simulink model "flanger"  (R2019a)
settings: Solver=FixedStepDiscrete  StartTime=0.0  StopTime=stop_time  RelTol=1e-3
InitFcn:
  | sm_callback_init
StopFcn:
  | sm_callback_stop
values from neighbouring files (symbols this model uses):
  mp = sm_init_avalon_signals(mp)    [sm_callback_init.m]
libraries: simulink x3, dspsigops x2
settings Model: Creator=Ross  LastModifiedBy=bugsbunny
settings DataIOCC: ReturnWorkspaceOutputs=off
settings OptimizationCC: BlockReduction=off  ConditionallyExecuteInputs=off  DefaultParameterBehavior=Inlined
settings DebuggingCC: ReadBeforeWriteMsg=DisableAll  WriteAfterWriteMsg=DisableAll  WriteAfterReadMsg=DisableAll  AlgebraicLoopMsg=error  MultiTaskDSMMsg=none  SingleTaskRateTransMsg=error  PregeneratedLibrarySubsystemCodeDiagnostic=none  ArithmeticOperatorsInVariantConditions=warning
settings HardwareCC: ProdBitPerPointer=32  ProdBitPerSizeT=32  ProdBitPerPtrDiffT=32  ProdLargestAtomicFloat=None  ProdIntDivRoundTo=Undefined  ProdEndianess=Unspecified  ProdWordSize=32  ProdHWDeviceType=ASIC/FPGA->ASIC/FPGA  TargetBitPerPointer=64  TargetBitPerSizeT=64  TargetBitPerPtrDiffT=64  TargetLongLongMode=on  TargetIntDivRoundTo=Zero  TargetEndianess=LittleEndian  TargetWordSize=64  TargetHWDeviceType=Custom Processor->MATLAB Host Computer  ProdEqTarget=off
settings ModelReferenceCC: UpdateModelReferenceTargets=IfOutOfDate
settings SFSimCC: SFSimEcho=off  SimUseLocalCustomCode=off
settings RTWCC: RTWUseLocalCustomCode=off

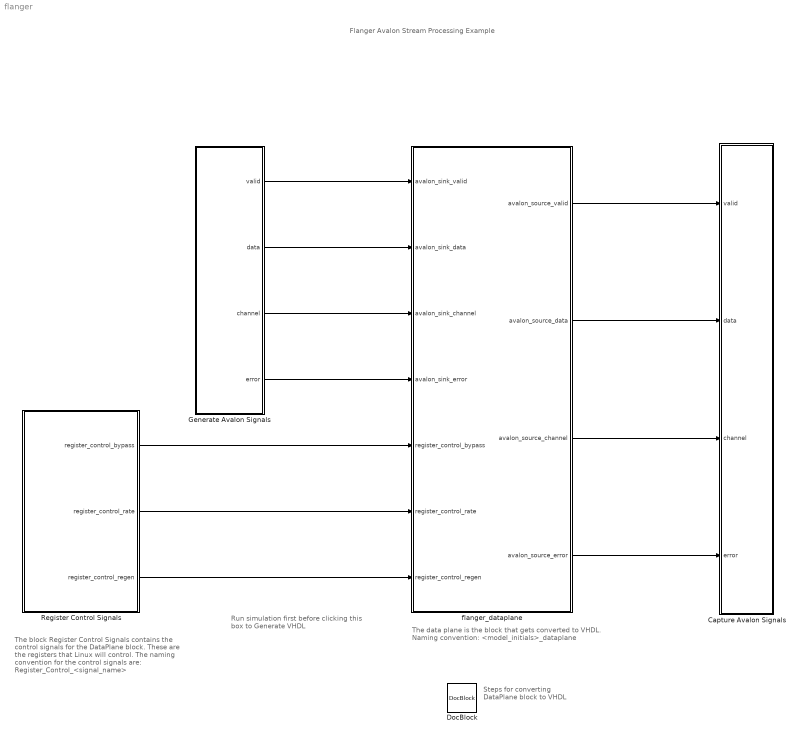
== system flanger ==
  note: The data plane is the block that gets converted to VHDL. Naming convention: <model_initials>_dataplane
  note: Steps for converting
      | DataPlane block
      | to VHDL
  note: Flanger
      | Avalon Stream Processing Example
  note: Run simulation first
      | before clicking this box to
      | Generate VHDL
  note: The block Register Control Signals contains
      | the control signals for the DataPlane block.
      | These are the registers that Linux will control.
      | The naming convention for the control
      | signals are:  Register_Control_<signal_name>
  Capture Avalon Signals : Subsystem
  DocBlock : simulink/Model-Wide Utilities/DocBlock  DocumentType=HTML
  Generate Avalon Signals : Subsystem
  Register Control Signals : Subsystem
  flanger_dataplane : Subsystem  TreatAsAtomicUnit=on
  wires:
  Generate Avalon Signals/2(data) -> flanger_dataplane/2(avalon_sink_data)
  Generate Avalon Signals/1(valid) -> flanger_dataplane/1(avalon_sink_valid)
  Generate Avalon Signals/3(channel) -> flanger_dataplane/3(avalon_sink_channel)
  Generate Avalon Signals/4(error) -> flanger_dataplane/4(avalon_sink_error)
  flanger_dataplane/2(avalon_source_data) -> Capture Avalon Signals/2(data)
  flanger_dataplane/1(avalon_source_valid) -> Capture Avalon Signals/1(valid)
  flanger_dataplane/3(avalon_source_channel) -> Capture Avalon Signals/3(channel)
  flanger_dataplane/4(avalon_source_error) -> Capture Avalon Signals/4(error)
  Register Control Signals/1(register_control_bypass) -> flanger_dataplane/5(register_control_bypass)
  Register Control Signals/2(register_control_rate) -> flanger_dataplane/6(register_control_rate)
  Register Control Signals/3(register_control_regen) -> flanger_dataplane/7(register_control_regen)

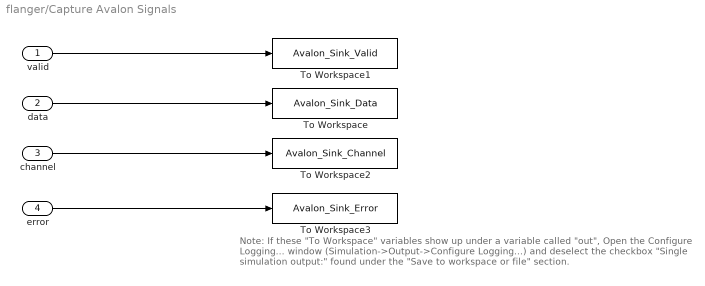
== system flanger/Capture Avalon Signals ==
  note: Note:  If these "To Workspace" variables show up under a variable called "out",
      | Open the Configure Logging... window (Simulation->Output->Configure Logging...)
      | and deselect the checkbox "Single simulation output:" found under the "Save to workspace or file" section.
  valid : Inport
  data : Inport  Port=2
  channel : Inport  Port=3
  error : Inport  Port=4
  To Workspace : ToWorkspace  VariableName=Avalon_Sink_Data  SaveFormat=Timeseries  SampleTime=-1
  To Workspace1 : ToWorkspace  VariableName=Avalon_Sink_Valid  SaveFormat=Timeseries  SampleTime=-1
  To Workspace2 : ToWorkspace  VariableName=Avalon_Sink_Channel  SaveFormat=Timeseries  SampleTime=-1
  To Workspace3 : ToWorkspace  VariableName=Avalon_Sink_Error  SaveFormat=Timeseries  SampleTime=-1
  wires:
  data/1 -> To Workspace/1
  valid/1 -> To Workspace1/1
  error/1 -> To Workspace3/1
  channel/1 -> To Workspace2/1

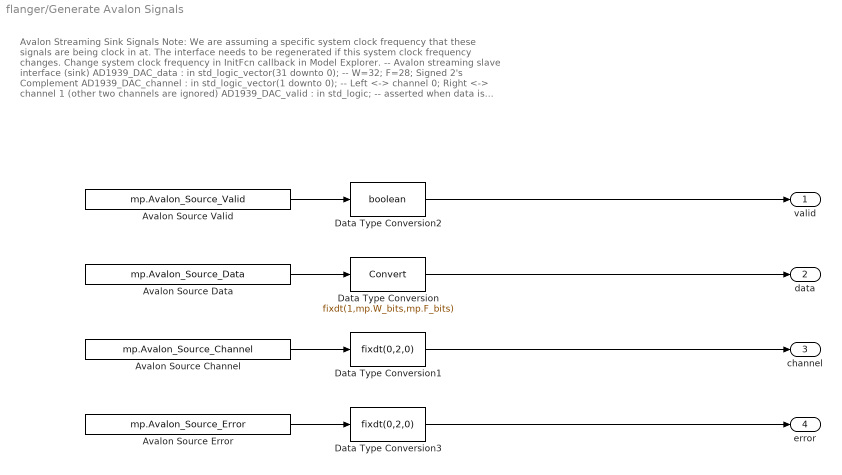
== system flanger/Generate Avalon Signals ==
  note: Avalon Streaming Sink Signals
      | Note: We are assuming a specific system clock frequency that these signals are being clock in at.
      | The interface needs to be regenerated if this system clock frequency changes. Change system clock frequency in InitFcn callback in Model Explorer.
      |
      | -- Avalon streaming slave interface (sink)
      | AD1939_DAC_data : in std_logic_vector(31 downto 0); -- W=32; F=28; Signed 2's Complement
      | AD1939_DAC_channel : in std_logic_vector(1 downto 0); -- Left <-> channel 0; Right <-> channel 1 (other two channels are ignored)
      | AD1939_DAC_valid : in std_logic; -- asserted when data is valid
      | AD1939_DAC_error : in std_logic_vector(1 downto 0) -- error channel is ignored, assumed to be error free at this point
      |
      | For more information on the data-channel-valid protocol, s ee chapter 5 in Intel's Avalon Interfaced Specification (p. 40) at https://www.intel.com/content/dam/www/programmable/us/en/pdfs/literature/manual/mnl_avalon_spec.pdf
  Avalon Source Channel : FromWorkspace  VariableName=mp.Avalon_Source_Channel  OutDataTypeStr=double  SampleTime=mp.Ts_system
  "Avalon Source Data " : FromWorkspace  VariableName=mp.Avalon_Source_Data  OutDataTypeStr=double  SampleTime=mp.Ts_system
  Avalon Source Error : FromWorkspace  VariableName=mp.Avalon_Source_Error  OutDataTypeStr=double  SampleTime=mp.Ts_system
  Avalon Source Valid : FromWorkspace  VariableName=mp.Avalon_Source_Valid  OutDataTypeStr=double  SampleTime=mp.Ts_system
  Data Type Conversion : DataTypeConversion  OutDataTypeStr=fixdt(1,mp.W_bits,mp.F_bits)
  Data Type Conversion1 : DataTypeConversion  OutDataTypeStr=fixdt(0,2,0)
  Data Type Conversion2 : DataTypeConversion  OutDataTypeStr=boolean
  Data Type Conversion3 : DataTypeConversion  OutDataTypeStr=fixdt(0,2,0)
  valid : Outport
  data : Outport  Port=2
  channel : Outport  Port=3
  error : Outport  Port=4
  wires:
  Data Type Conversion1/1 -> channel/1
  Data Type Conversion2/1 -> valid/1
  Avalon Source Error/1 -> Data Type Conversion3/1
  Data Type Conversion/1 -> data/1
  Avalon Source Valid/1 -> Data Type Conversion2/1
  Data Type Conversion3/1 -> error/1
  Avalon Source Channel/1 -> Data Type Conversion1/1
  "Avalon Source Data "/1 -> Data Type Conversion/1

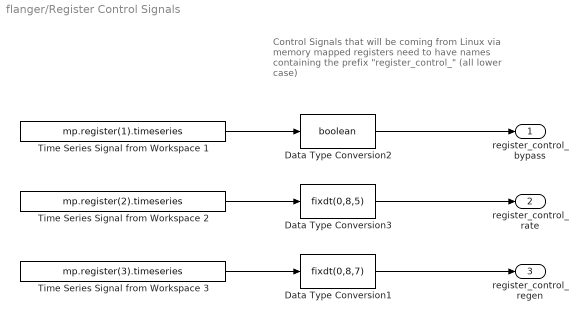
== system flanger/Register Control Signals ==
  note: Control Signals that will be coming from Linux via
      | memory mapped registers need to have names
      | containing the prefix "register_control_"
      | (all lower case)
  Data Type Conversion1 : DataTypeConversion  OutDataTypeStr=fixdt(0,8,7)
  Data Type Conversion2 : DataTypeConversion  OutDataTypeStr=boolean
  Data Type Conversion3 : DataTypeConversion  OutDataTypeStr=fixdt(0,8,5)
  Time Series Signal from Workspace 1 : FromWorkspace  VariableName=mp.register(1).timeseries  OutDataTypeStr=double  SampleTime=mp.Ts_system
  Time Series Signal from Workspace 2 : FromWorkspace  VariableName=mp.register(2).timeseries  OutDataTypeStr=double  SampleTime=mp.Ts_system
  Time Series Signal from Workspace 3 : FromWorkspace  VariableName=mp.register(3).timeseries  OutDataTypeStr=double  SampleTime=mp.Ts_system
  register_control_bypass : Outport
  register_control_rate : Outport  Port=2
  register_control_regen : Outport  Port=3
  wires:
  Time Series Signal from Workspace 1/1 -> Data Type Conversion2/1
  Data Type Conversion2/1 -> register_control_bypass/1
  Time Series Signal from Workspace 2/1 -> Data Type Conversion3/1
  Data Type Conversion3/1 -> register_control_rate/1
  Time Series Signal from Workspace 3/1 -> Data Type Conversion1/1
  Data Type Conversion1/1 -> register_control_regen/1

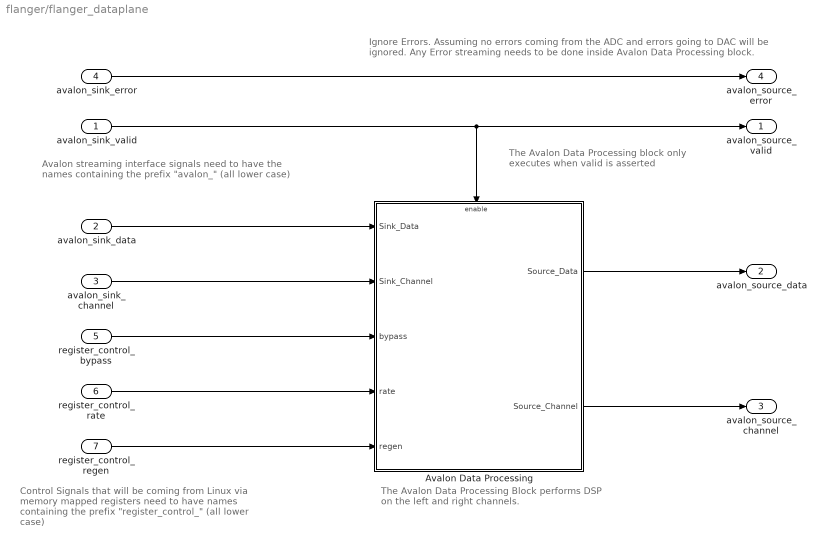
== system flanger/flanger_dataplane ==
  note: Control Signals that will be coming from Linux via
      | memory mapped registers need to have names
      | containing the prefix "register_control_"
      | (all lower case)
  note: The Avalon Data Processing Block
      | performs DSP on the left and right channels.
  note: The Avalon Data Processing block
      | only executes when valid is asserted
  note: Ignore Errors.
      | Assuming no errors coming from the ADC and errors going to DAC will be ignored.
      | Any Error streaming needs to be done inside Avalon Data Processing block.
  note: Avalon streaming interface signals need to have the
      | names containing the prefix "avalon_"
      | (all lower case)
  avalon_sink_valid : Inport
  avalon_sink_data : Inport  Port=2
  avalon_sink_channel : Inport  Port=3
  avalon_sink_error : Inport  Port=4
  register_control_bypass : Inport  Port=5
  register_control_rate : Inport  Port=6
  register_control_regen : Inport  Port=7
  Avalon Data Processing : Subsystem  TreatAsAtomicUnit=on
  avalon_source_valid : Outport
  avalon_source_data : Outport  Port=2
  avalon_source_channel : Outport  Port=3
  avalon_source_error : Outport  Port=4
  wires:
  avalon_sink_channel/1 -> Avalon Data Processing/2(Sink_Channel)
  avalon_sink_error/1 -> avalon_source_error/1
  Avalon Data Processing/1(Source_Data) -> avalon_source_data/1
  avalon_sink_valid/1 -> avalon_source_valid/1, Avalon Data Processing/Enable
  avalon_sink_data/1 -> Avalon Data Processing/1(Sink_Data)
  Avalon Data Processing/2(Source_Channel) -> avalon_source_channel/1
  register_control_bypass/1 -> Avalon Data Processing/3(bypass)
  register_control_rate/1 -> Avalon Data Processing/4(rate)
  register_control_regen/1 -> Avalon Data Processing/5(regen)

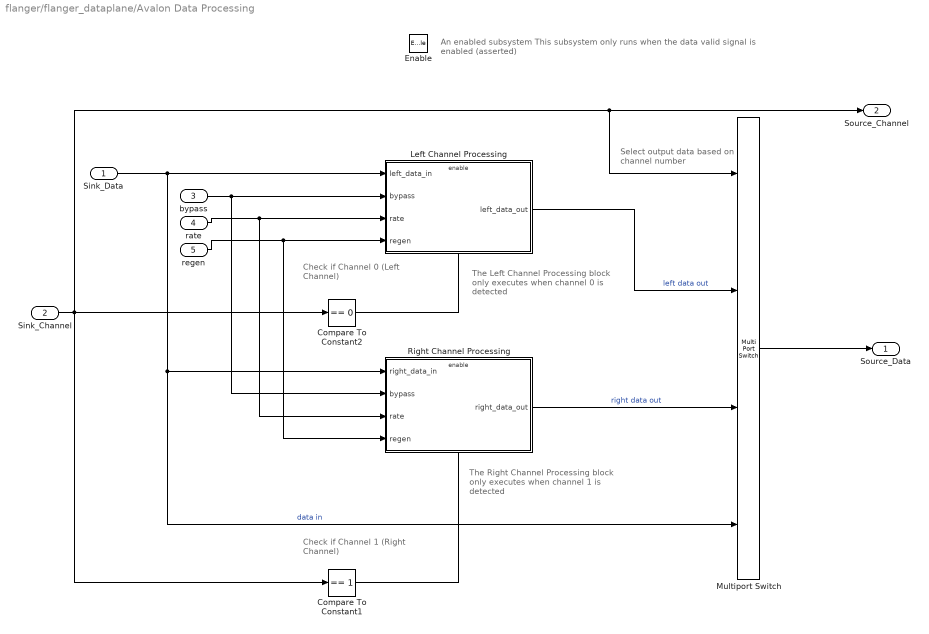
== system flanger/flanger_dataplane/Avalon Data Processing ==
  note: Select output data
      | based on channel number
  note: Check if Channel 0
      | (Left Channel)
  note: The Left Channel Processing block
      | only executes when channel 0
      | is detected
  note: The Right Channel Processing block
      | only executes when channel 1
      | is detected
  note: Check if Channel 1
      | (Right Channel)
  note: An enabled subsystem
      | This subsystem only runs when the data valid signal is enabled (asserted)
  Sink_Data : Inport
  Sink_Channel : Inport  Port=2
  bypass : Inport  Port=3
  rate : Inport  Port=4
  regen : Inport  Port=5
  Enable : EnablePort
  Compare To Constant1 : simulink/Logic and Bit Operations/Compare To Constant  relop===  const=1  OutDataTypeStr=boolean
  Compare To Constant2 : simulink/Logic and Bit Operations/Compare To Constant  relop===  const=0  OutDataTypeStr=boolean
  Left Channel Processing : Subsystem  TreatAsAtomicUnit=on
  Multiport Switch : MultiPortSwitch  DataPortOrder=Zero-based contiguous  zeroidx=on
  Right Channel Processing : Subsystem  TreatAsAtomicUnit=on
  Source_Data : Outport  InitialOutput=0
  Source_Channel : Outport  Port=2  InitialOutput=0
  wires:
  Sink_Channel/1 -> Compare To Constant1/1, Compare To Constant2/1, Source_Channel/1, Multiport Switch/1
  Compare To Constant2/1 -> Left Channel Processing/Enable
  Sink_Data/1 -> Left Channel Processing/1(left_data_in), Multiport Switch/4, Right Channel Processing/1(right_data_in)  "data in"
  Left Channel Processing/1(left_data_out) -> Multiport Switch/2  "left data out"
  Right Channel Processing/1(right_data_out) -> Multiport Switch/3  "right data out"
  Multiport Switch/1 -> Source_Data/1
  rate/1 -> Right Channel Processing/3(rate), Left Channel Processing/3(rate)
  regen/1 -> Right Channel Processing/4(regen), Left Channel Processing/4(regen)
  bypass/1 -> Right Channel Processing/2(bypass), Left Channel Processing/2(bypass)
  Compare To Constant1/1 -> Right Channel Processing/Enable

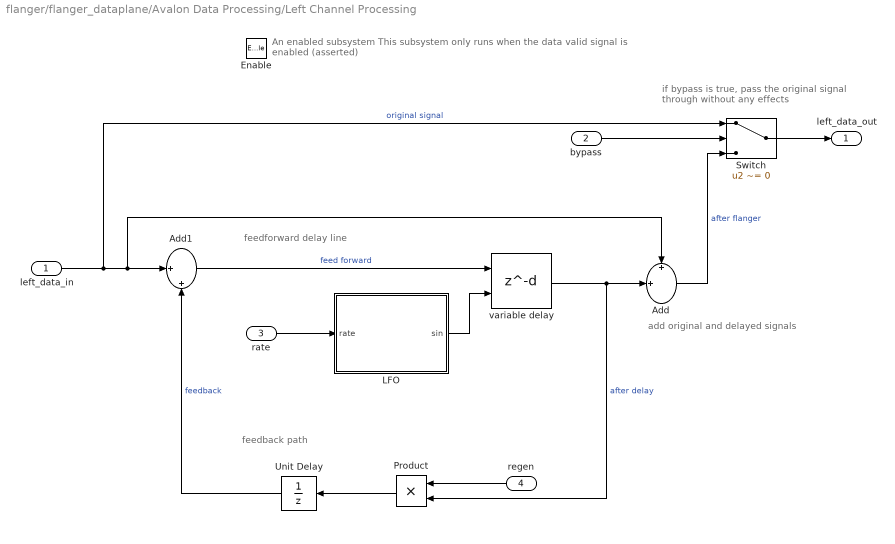
== system flanger/flanger_dataplane/Avalon Data Processing/Left Channel Processing ==
  note: if bypass is true, pass the original signal
      | through without any effects
  note: add original and delayed signals
  note: feedforward delay line
  note: feedback path
  note: An enabled subsystem
      | This subsystem only runs when the data valid signal is enabled (asserted)
  left_data_in : Inport
  bypass : Inport  Port=2
  rate : Inport  Port=3
  regen : Inport  Port=4
  Enable : EnablePort
  Add : Sum  Inputs=+|+||  OutDataTypeStr=fixdt(mp.signed, mp.W_bits, mp.F_bits)
  Add1 : Sum  Inputs=||+|+  OutDataTypeStr=fixdt(1, 40, 32)
  LFO : Subsystem
  Product : Product  OutDataTypeStr=Inherit: Inherit via back propagation
  Switch : Switch  Criteria=u2 ~= 0
  Unit Delay : UnitDelay  SampleTime=-1  HasFrameUpgradeWarning=on
  variable delay : Delay  DelayLengthSource=Input port  DelayLength=1  DelayLengthUpperLimit=mp.delay_max  InitialCondition=0  DiagnosticForDelayLength=Error  UseCircularBuffer=on
      settings: InputPortMap=u0,p1
  left_data_out : Outport  InitialOutput=0
  wires:
  left_data_in/1 -> Switch/1, Add1/1, Add/1  "original signal"
  Add/1 -> Switch/3  "after flanger"
  Switch/1 -> left_data_out/1
  bypass/1 -> Switch/2
  LFO/1(sin) -> variable delay/2
  rate/1 -> LFO/1(rate)
  variable delay/1 -> Add/2, Product/2  "after delay"
  regen/1 -> Product/1
  Product/1 -> Unit Delay/1
  Add1/1 -> variable delay/1  "feed forward"
  Unit Delay/1 -> Add1/2  "feedback"

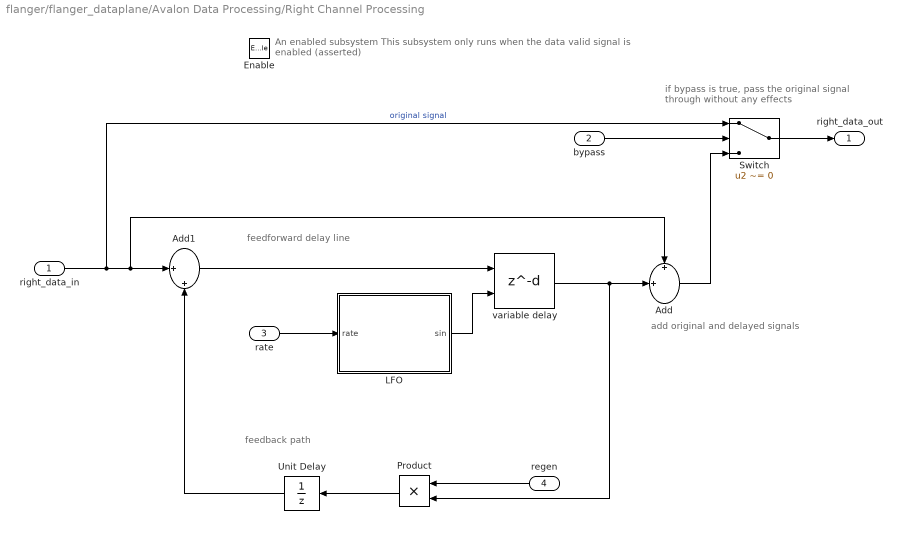
== system flanger/flanger_dataplane/Avalon Data Processing/Right Channel Processing ==
  note: feedforward delay line
  note: feedback path
  note: add original and delayed signals
  note: if bypass is true, pass the original signal
      | through without any effects
  note: An enabled subsystem
      | This subsystem only runs when the data valid signal is enabled (asserted)
  right_data_in : Inport
  bypass : Inport  Port=2
  rate : Inport  Port=3
  regen : Inport  Port=4
  Enable : EnablePort
  Add : Sum  Inputs=+|+||  OutDataTypeStr=fixdt(mp.signed, mp.W_bits, mp.F_bits)
  Add1 : Sum  Inputs=||+|+  OutDataTypeStr=fixdt(1, 40, 32)
  LFO : Subsystem
  Product : Product  OutDataTypeStr=Inherit: Inherit via back propagation
  Switch : Switch  Criteria=u2 ~= 0
  Unit Delay : UnitDelay  SampleTime=-1  HasFrameUpgradeWarning=on
  variable delay : Delay  DelayLengthSource=Input port  DelayLength=1  DelayLengthUpperLimit=mp.delay_max  InitialCondition=0  DiagnosticForDelayLength=Error  UseCircularBuffer=on
      settings: InputPortMap=u0,p1
  right_data_out : Outport  InitialOutput=0
  wires:
  Unit Delay/1 -> Add1/2
  rate/1 -> LFO/1(rate)
  variable delay/1 -> Add/2, Product/2
  Add/1 -> Switch/3
  Switch/1 -> right_data_out/1
  bypass/1 -> Switch/2
  Product/1 -> Unit Delay/1
  Add1/1 -> variable delay/1
  regen/1 -> Product/1
  right_data_in/1 -> Switch/1, Add1/1, Add/1  "original signal"
  LFO/1(sin) -> variable delay/2

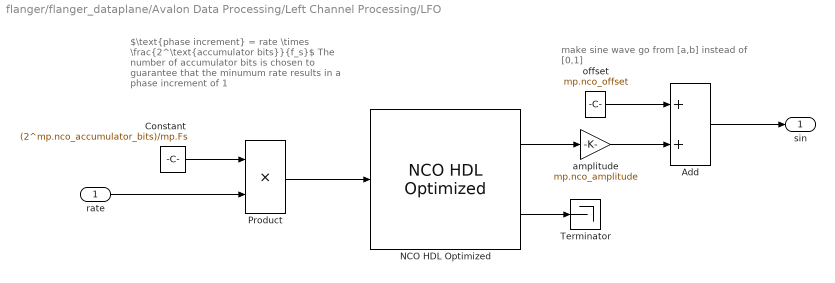
== system flanger/flanger_dataplane/Avalon Data Processing/Left Channel Processing/LFO ==
  note: $\text{phase increment} = rate \times \frac{2^\text{accumulator bits}}{f_s}$
      | The number of accumulator bits is chosen to guarantee that the minumum rate results in a phase increment of 1
  note: make sine wave go from [a,b]
      | instead of [0,1]
  rate : Inport
  Add : Sum
  Constant : Constant  Value=(2^mp.nco_accumulator_bits)/mp.Fs  OutDataTypeStr=fixdt(0,16,12)  SampleTime=-1
  NCO HDL Optimized : dspsigops/NCO HDL Optimized  PhaseIncrementSource=Input port  PhaseIncrement=100  PhaseOffsetSource=Property  PhaseOffset=0  DitherSource=Property  NumDitherBits=mp.nco_dither_bits  PhaseQuantization=on  NumQuantizerAccumulatorBits=mp.nco_quantizer_bits  LUTCompress=on  ResetAction=off  ValidInputPort=off  Waveform=Sine  PhasePort=off  SimulateUsing=Code generation  AccumulatorWL=mp.nco_accumulator_bits  OutputDataType=Binary point scaling  OutputWL=16  OutputFL=14
      settings: SourceProductName=DSP System Toolbox  SourceProductBaseCode=DS
  Product : Product
  Terminator : Terminator
  amplitude : Gain  Gain=mp.nco_amplitude  OutDataTypeStr=int16
  offset : Constant  Value=mp.nco_offset  OutDataTypeStr=uint16  SampleTime=-1
  sin : Outport
  wires:
  Product/1 -> NCO HDL Optimized/1
  rate/1 -> Product/2
  Constant/1 -> Product/1
  NCO HDL Optimized/1 -> amplitude/1
  amplitude/1 -> Add/2
  offset/1 -> Add/1
  Add/1 -> sin/1
  NCO HDL Optimized/2 -> Terminator/1

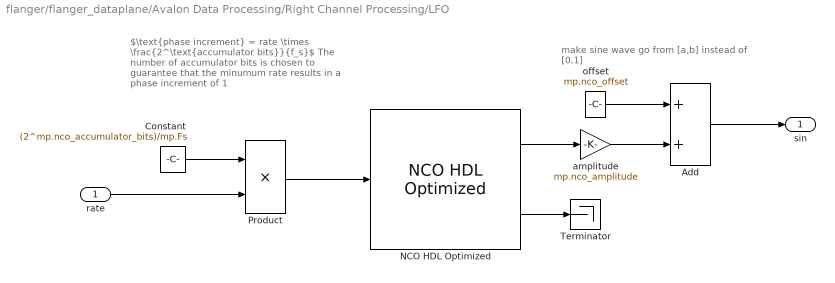
== system flanger/flanger_dataplane/Avalon Data Processing/Right Channel Processing/LFO ==
  note: make sine wave go from [a,b]
      | instead of [0,1]
  note: $\text{phase increment} = rate \times \frac{2^\text{accumulator bits}}{f_s}$
      | The number of accumulator bits is chosen to guarantee that the minumum rate results in a phase increment of 1
  rate : Inport
  Add : Sum
  Constant : Constant  Value=(2^mp.nco_accumulator_bits)/mp.Fs  OutDataTypeStr=fixdt(0,16,12)  SampleTime=-1
  NCO HDL Optimized : dspsigops/NCO HDL Optimized  PhaseIncrementSource=Input port  PhaseIncrement=100  PhaseOffsetSource=Property  PhaseOffset=0  DitherSource=Property  NumDitherBits=mp.nco_dither_bits  PhaseQuantization=on  NumQuantizerAccumulatorBits=mp.nco_quantizer_bits  LUTCompress=on  ResetAction=off  ValidInputPort=off  Waveform=Sine  PhasePort=off  SimulateUsing=Code generation  AccumulatorWL=mp.nco_accumulator_bits  OutputDataType=Binary point scaling  OutputWL=16  OutputFL=14
      settings: SourceProductName=DSP System Toolbox  SourceProductBaseCode=DS
  Product : Product
  Terminator : Terminator
  amplitude : Gain  Gain=mp.nco_amplitude  OutDataTypeStr=int16
  offset : Constant  Value=mp.nco_offset  OutDataTypeStr=uint16  SampleTime=-1
  sin : Outport
  wires:
  NCO HDL Optimized/2 -> Terminator/1
  amplitude/1 -> Add/2
  rate/1 -> Product/2
  offset/1 -> Add/1
  Product/1 -> NCO HDL Optimized/1
  Add/1 -> sin/1
  Constant/1 -> Product/1
  NCO HDL Optimized/1 -> amplitude/1
